simulink model "PFC_SIL_model"  (R2021a)
settings: Solver=VariableStepAuto  StartTime=0.0  StopTime=1  MaxStep=1e-5  RelTol=1e-3
values from neighbouring files (symbols this model uses):
  ki_current = 140/3    (= 46.6666666667)    [PFC_drscrete.m]
  ki_volt = 0.4    [PFC_drscrete.m]
  kp_curr = 0.027    [PFC_drscrete.m]
  kp_volt = 0.03    [PFC_drscrete.m]
  Po = 15000/3    (= 5000)    [PFC_drscrete.m]
  Ramp = 0.008    [PFC_drscrete.m]
  ramp_initial = 0.2    [PFC_drscrete.m]
  ramp_sat_max = 0.95    [PFC_drscrete.m]
  ramp_sat_min = 0.2    [PFC_drscrete.m]
  Ro = 100e3    (= 100000)    [PFC_drscrete.m]
  Softstart_th = 30    [PFC_drscrete.m]
  Vm = 400    [PFC_drscrete.m]
  Vo = 100    [PFC_drscrete.m]
undefined symbols (not defined in the file or in its folder): DiscIntNeverNeededParam, T_Finished, T_step
libraries: spsSeriesRLCBranchLib x34, simulink x19, spsMosfetLib x8, spsPWMGeneratorDCDCLib x8, spsControlledVoltageSourceLib x6, spsGroundLib x6, spsVoltageMeasurementLib x6, spsCurrentMeasurementLib x3, pid_lib x2, spsDiodeLib x2, spspowerguiLib x1
(part 2 of 2)

== system PFC_SIL_model/Subsystem/Subsystem5/Subsystem4/Soft Switch 1/Normal operation  ==
  PID output : Inport
  AC/ input : Inport  Port=2
  Enable : EnablePort
  Constant : Constant
  Constant1 : Constant  Value=0
  Constant2 : Constant
  Constant3 : Constant
  Constant4 : Constant  Value=0
  Data Store Write3 : DataStoreWrite  DataStoreName=Start_STOP_TIMER  IndexOptions=Index vector (dialog)  Indices=1  OutputSizes=1
  Subtract : Sum  Inputs=-+
  Subtract1 : Sum  Inputs=-+
  Switch : Switch  Criteria=u2 > Threshold
  Outport : Outport
  Outport1 : Outport  Port=2
  Outport2 : Outport  Port=3
  Outport3 : Outport  Port=4
  wires:
  Constant4/1 -> Data Store Write3/1
  PID output/1 -> Outport2/1, Subtract1/1
  Constant3/1 -> Subtract1/2
  Constant1/1 -> Switch/3
  Constant2/1 -> Subtract/2
  Constant/1 -> Switch/1
  AC/ input/1 -> Switch/2
  Switch/1 -> Subtract/1, Outport/1
  Subtract/1 -> Outport1/1
  Subtract1/1 -> Outport3/1

== system PFC_SIL_model/Subsystem/Subsystem5/Subsystem4/Soft Switch 1/Outout Ramp 1 ==
  Enable : Inport
  Constant1 : Constant  Value=0.0082
  Ramp Generator : Subsystem
  Saturation : Saturate  UpperLimit=1  LowerLimit=0
  Outport : Outport
  wires:
  Saturation/1 -> Outport/1
  Ramp Generator/1(Ramp) -> Saturation/1
  Constant1/1 -> Ramp Generator/1(Ramp_Time)
  Enable/1 -> Ramp Generator/2(Enable)

== system PFC_SIL_model/Subsystem/Subsystem5/Subsystem4/Soft Switch 1/Positive to negative subsystem  ==
  Inport : Inport
  Enable : EnablePort
  Constant : Constant
  Constant16 : Constant  Value=0
  Constant17 : Constant  Value=0
  Constant18 : Constant  Value=0
  Data Store Write2 : DataStoreWrite  DataStoreName=Start_STOP_TIMER  IndexOptions=Index vector (dialog)  Indices=1  OutputSizes=1
  Outport : Outport
  Outport1 : Outport  Port=2
  Outport2 : Outport  Port=3
  Outport3 : Outport  Port=4
  wires:
  Constant18/1 -> Outport1/1
  Constant17/1 -> Outport3/1
  Constant16/1 -> Outport/1
  Inport/1 -> Outport2/1
  Constant/1 -> Data Store Write2/1

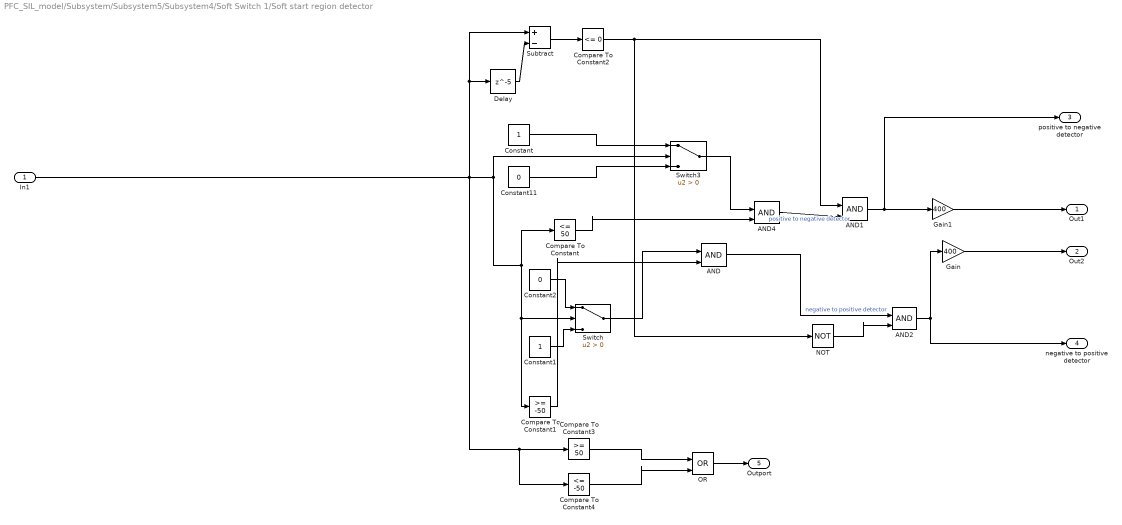
== system PFC_SIL_model/Subsystem/Subsystem5/Subsystem4/Soft Switch 1/Soft start region detector  ==
  In1 : Inport
  AND{,1..2,4} (4 alike) : Logic  IconShape=distinctive  AllPortsSameDT=off  OutDataTypeStr=boolean
  Compare To Constant : simulink/Logic and Bit Operations/Compare To Constant  relop=<=  const=50  OutDataTypeStr=boolean
  Compare To Constant1 : simulink/Logic and Bit Operations/Compare To Constant  relop=>=  const=-50  OutDataTypeStr=boolean
  Compare To Constant2 : simulink/Logic and Bit Operations/Compare To Constant  relop=<=  const=0  OutDataTypeStr=boolean
  Compare To Constant3 : simulink/Logic and Bit Operations/Compare To Constant  relop=>=  const=50  OutDataTypeStr=boolean
  Compare To Constant4 : simulink/Logic and Bit Operations/Compare To Constant  relop=<=  const=-50  OutDataTypeStr=boolean
  Constant : Constant
  Constant1 : Constant
  Constant11 : Constant  Value=0
  Constant2 : Constant  Value=0
  Delay : Delay  DelayLength=5
  Gain : Gain  Gain=400
  Gain1 : Gain  Gain=400
  NOT : Logic  Operator=NOT  IconShape=distinctive  AllPortsSameDT=off  OutDataTypeStr=boolean
  OR : Logic  Operator=OR  IconShape=distinctive  AllPortsSameDT=off  OutDataTypeStr=boolean
  Subtract : Sum  Inputs=+-
  Switch : Switch  Criteria=u2 > Threshold
  Switch3 : Switch  Criteria=u2 > Threshold
  Out1 : Outport
  Out2 : Outport  Port=2
  positive to negative detector : Outport  Port=3
  negative to positive detector : Outport  Port=4
  Outport : Outport  Port=5
  wires:
  AND4/1 -> AND1/2  "positive to negative detector"
  Constant11/1 -> Switch3/3
  In1/1 -> Compare To Constant4/1, Compare To Constant3/1, Delay/1, Subtract/1, Switch3/2, Compare To Constant1/1, Switch/2, Compare To Constant/1
  Compare To Constant/1 -> AND4/2
  AND/1 -> AND2/1  "negative to positive detector"
  Switch3/1 -> AND4/1
  Constant/1 -> Switch3/1
  Gain1/1 -> Out1/1
  Gain/1 -> Out2/1
  Constant1/1 -> Switch/3
  Constant2/1 -> Switch/1
  Switch/1 -> AND/1
  Compare To Constant1/1 -> AND/2
  Delay/1 -> Subtract/2
  Subtract/1 -> Compare To Constant2/1
  Compare To Constant2/1 -> NOT/1, AND1/1
  NOT/1 -> AND2/2
  AND2/1 -> negative to positive detector/1, Gain/1
  AND1/1 -> positive to negative detector/1, Gain1/1
  Compare To Constant3/1 -> OR/1
  Compare To Constant4/1 -> OR/2
  OR/1 -> Outport/1

== system PFC_SIL_model/Subsystem/Subsystem5/Subsystem4/Soft Switch 1/Timer ==
  In1 : Inport
  Constant : Constant  Value=0
  Constant1 : Constant  Value=T_step
  Constant3 : Constant  Value=0
  Constant4 : Constant
  Saturation : Saturate  UpperLimit=1  LowerLimit=0
  Scope1 : Scope
  Sum : Sum  Inputs=|++
  Switch : Switch  Criteria=u2 > Threshold
  Switch1 : Switch  Threshold=T_Finished
  Terminator : Terminator
  Unit Delay : UnitDelay  SampleTime=-1  HasFrameUpgradeWarning=on
  Outport : Outport
  wires:
  Switch/1 -> Scope1/1, Saturation/1, Switch1/2, Unit Delay/1
  Constant1/1 -> Sum/2
  Constant/1 -> Switch/3
  Unit Delay/1 -> Sum/1
  Constant3/1 -> Switch1/3
  Sum/1 -> Switch/1
  Constant4/1 -> Switch1/1
  In1/1 -> Switch/2
  Switch1/1 -> Terminator/1
  Saturation/1 -> Outport/1

== system PFC_SIL_model/Subsystem/Subsystem5/Subsystem4/Soft Switch 1/negative to positive subsystem  ==
  Inport : Inport
  Enable : EnablePort
  Constant : Constant  Commented=on  Value=0
  Constant12 : Constant  Value=0
  Constant13 : Constant  Value=0
  Constant14 : Constant  Value=0
  Constant2 : Constant
  Constant3 : Constant  Commented=on  Value=T_step
  Data Store Write2 : DataStoreWrite  DataStoreName=Start_STOP_TIMER  IndexOptions=Index vector (dialog)  Indices=1  OutputSizes=1
  Saturation1 : Saturate  Commented=on
  Sum : Sum  Commented=on  Inputs=|++
  Switch : Switch  Commented=on  Criteria=u2 > Threshold
  Unit Delay : UnitDelay  Commented=on  SampleTime=-1  HasFrameUpgradeWarning=on
  Outport : Outport
  Outport1 : Outport  Port=2
  Outport2 : Outport  Port=3
  Outport3 : Outport  Port=4
  wires:
  Constant13/1 -> Outport2/1
  Constant12/1 -> Outport/1
  Constant14/1 -> Outport1/1
  Inport/1 -> Outport3/1
  Constant2/1 -> Data Store Write2/1
  Unit Delay/1 -> Sum/1
  Constant/1 -> Switch/3
  Sum/1 -> Switch/1
  Switch/1 -> Unit Delay/1
  Constant3/1 -> Sum/2
  ? -> Switch/2

== system PFC_SIL_model/Subsystem/Subsystem5/Subsystem3/Soft Switch 1/Ramp up /Ramp Generator ==
  Ramp_Time : Inport
  Enable : Inport  Port=2
  Divide : Product  Inputs=*/  RndMeth=Simplest  OutDataTypeStr=Inherit: Same as first input
  NOT : Logic  Operator=NOT  IconShape=distinctive  AllPortsSameDT=off  OutDataTypeStr=boolean
  One : Constant  SampleTime=-1
  Ramp Generator : DiscreteIntegrator  IntegratorMethod=Accumulation: Forward Euler  gainval=1  ExternalReset=sampled level  InitialCondition=ramp_initial  SampleTime=-1  RndMeth=Simplest  LimitOutput=on  UpperSaturationLimit=1  LowerSaturationLimit=0  ICPrevOutput=DiscIntNeverNeededParam  ICPrevScaledInput=DiscIntNeverNeededParam
  Sample_Time : Gain  Gain=0.00001  RndMeth=Simplest  OutDataTypeStr=Inherit: Same as input
  Ramp : Outport
  wires:
  Divide/1 -> Sample_Time/1
  Ramp Generator/1 -> Ramp/1  "Eps"
  Sample_Time/1 -> Ramp Generator/1
  One/1 -> Divide/1
  Ramp_Time/1 -> Divide/2
  Enable/1 -> NOT/1
  NOT/1 -> Ramp Generator/2

== system PFC_SIL_model/Subsystem/Subsystem5/Subsystem3/Soft Switch 1/ramp down/Ramp Generator ==
  Ramp_Time : Inport
  Enable : Inport  Port=2
  Divide : Product  Inputs=*/  RndMeth=Simplest  OutDataTypeStr=Inherit: Same as first input
  NOT : Logic  Operator=NOT  IconShape=distinctive  AllPortsSameDT=off  OutDataTypeStr=boolean
  One : Constant  SampleTime=-1
  Ramp Generator : DiscreteIntegrator  IntegratorMethod=Accumulation: Forward Euler  gainval=1  ExternalReset=sampled level  InitialCondition=ramp_initial  SampleTime=-1  RndMeth=Simplest  LimitOutput=on  UpperSaturationLimit=1  LowerSaturationLimit=0  ICPrevOutput=DiscIntNeverNeededParam  ICPrevScaledInput=DiscIntNeverNeededParam
  Sample_Time : Gain  Gain=0.00001  RndMeth=Simplest  OutDataTypeStr=Inherit: Same as input
  Ramp : Outport
  wires:
  Divide/1 -> Sample_Time/1
  Ramp Generator/1 -> Ramp/1  "Eps"
  Sample_Time/1 -> Ramp Generator/1
  One/1 -> Divide/1
  Ramp_Time/1 -> Divide/2
  Enable/1 -> NOT/1
  NOT/1 -> Ramp Generator/2

== system PFC_SIL_model/Subsystem/Subsystem5/Subsystem4/Soft Switch 1/Outout Ramp 1/Ramp Generator ==
  Ramp_Time : Inport
  Enable : Inport  Port=2
  Divide : Product  Inputs=*/  RndMeth=Simplest  OutDataTypeStr=Inherit: Same as first input
  NOT : Logic  Operator=NOT  IconShape=distinctive  AllPortsSameDT=off  OutDataTypeStr=boolean
  One : Constant  SampleTime=-1
  Ramp Generator : DiscreteIntegrator  IntegratorMethod=Accumulation: Forward Euler  gainval=1  ExternalReset=sampled level  SampleTime=-1  RndMeth=Simplest  LimitOutput=on  UpperSaturationLimit=1  LowerSaturationLimit=0  ICPrevOutput=DiscIntNeverNeededParam  ICPrevScaledInput=DiscIntNeverNeededParam
  Sample_Time : Gain  Gain=0.00001  RndMeth=Simplest  OutDataTypeStr=Inherit: Same as input
  Ramp : Outport
  wires:
  Divide/1 -> Sample_Time/1
  Ramp Generator/1 -> Ramp/1  "Eps"
  Sample_Time/1 -> Ramp Generator/1
  One/1 -> Divide/1
  Ramp_Time/1 -> Divide/2
  Enable/1 -> NOT/1
  NOT/1 -> Ramp Generator/2
